simulink model "servo"  (R2015a)
settings: Solver=ode45  StartTime=0.0  StopTime=10.0  RelTol=1e-3
undefined symbols (not defined in the file): B, J, Kem, R
libraries: simulink x1
settings Model: Creator=root  LastModifiedBy=root

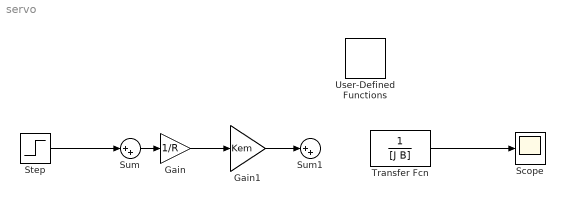
== system servo ==
  Gain : Gain  Gain=1/R
  Gain1 : Gain  Gain=Kem
  Scope : Scope
  Step : Step  SampleTime=0
  Sum : Sum  Inputs=|++
  Sum1 : Sum  Inputs=|++
  Transfer Fcn : TransferFcn  Denominator=[J B]
  User-Defined Functions : simulink/User-Defined Functions  SystemSampleTime=-1
      link override "MATLAB Function/ Demux ": Outputs=1
      link override "MATLAB Function/ SFunction ": FunctionName=sf_sfun
      link override MATLAB Function/u: Port=1
      link override MATLAB Function/y: Port=1
  wires:
  Step/1 -> Sum/1
  Sum/1 -> Gain/1
  Gain/1 -> Gain1/1
  Transfer Fcn/1 -> Scope/1
  Gain1/1 -> Sum1/1
  ? -> ?

== matlab function servo/User-Defined Functions/MATLAB Function ==
  data: u input; y output
function y = fcn(u)
%#codegen

y = u;
